simulink subsystem "MotoresPWM_Javi"  (R2023b)
settings: Solver=VariableStepAuto  StartTime=0.0  StopTime=10.0  RelTol=1e-3
libraries: arduinolib x6, simulink x2
settings Model: Creator=Usuario_UMA  LastModifiedBy=javie

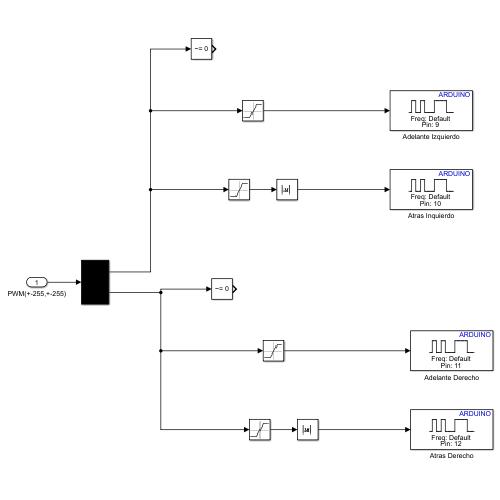
[thumbnail: Simulink's stored preview of the top-level diagram]
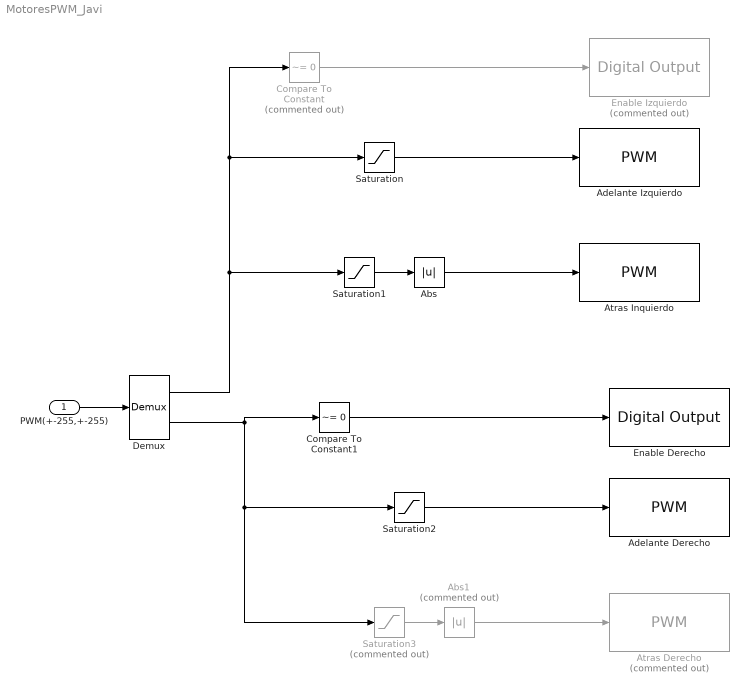
== system MotoresPWM_Javi ==
  PWM(+-255,+-255) : Inport
  Abs : Abs  SaturateOnIntegerOverflow=off
  Abs1 : Abs  Commented=on  SaturateOnIntegerOverflow=off
  Adelante Derecho : arduinolib/PWM  pinNumber=11  frequencyType=Default  desiredFrequency=490.2  achievableFrequency=490.2
  Adelante Izquierdo : arduinolib/PWM  pinNumber=9  frequencyType=Default  desiredFrequency=490.2  achievableFrequency=490.2
  Atras Derecho : arduinolib/PWM  Commented=on  pinNumber=12  frequencyType=Default  desiredFrequency=490.2  achievableFrequency=490.2
  Atras Inquierdo : arduinolib/PWM  pinNumber=10  frequencyType=Default  desiredFrequency=490.2  achievableFrequency=490.2
  Compare To Constant : simulink/Logic and Bit Operations/Compare To Constant  Commented=on  relop=~=  const=0  OutDataTypeStr=boolean
  Compare To Constant1 : simulink/Logic and Bit Operations/Compare To Constant  relop=~=  const=0  OutDataTypeStr=boolean
  Demux : Demux  Outputs=2
  Enable Derecho : arduinolib/Digital Output  pinNumber=7  Direction=output  blockPlatform=arduino
  Enable Izquierdo : arduinolib/Digital Output  Commented=on  pinNumber=6  Direction=output  blockPlatform=arduino
  Saturation : Saturate  UpperLimit=255  LowerLimit=1
  Saturation1 : Saturate  UpperLimit=-1  LowerLimit=-255
  Saturation2 : Saturate  UpperLimit=255  LowerLimit=1
  Saturation3 : Saturate  Commented=on  UpperLimit=-1  LowerLimit=-255
  wires:
  PWM(+-255,+-255)/1 -> Demux/1
  Abs/1 -> Atras Inquierdo/1
  Saturation/1 -> Adelante Izquierdo/1
  Saturation1/1 -> Abs/1
  Demux/1 -> Saturation1/1, Saturation/1, Compare To Constant/1
  Abs1/1 -> Atras Derecho/1
  Saturation3/1 -> Abs1/1
  Saturation2/1 -> Adelante Derecho/1
  Demux/2 -> Saturation3/1, Saturation2/1, Compare To Constant1/1
  Compare To Constant/1 -> Enable Izquierdo/1
  Compare To Constant1/1 -> Enable Derecho/1
